simulink model "DriverInLoopSpeedgoat"  (R2020b)
settings: Solver=ode3  StartTime=0.0  StopTime=inf  FixedStep=1e-3  RelTol=5e-3  EnableMultiTasking=on
StartFcn:
  | %tic
StopFcn:
  | %toc
model workspace (MAT data in the model file):
  A_mu = 10
  B_reff = 8.386
  Cz = 7766.25
  DCT_Param.Transmission.Ratios = [3.78 2.18 1.43 1.03 0.935 0.84]
  DCT_Param.Transmission.Shaft_Inertia_Odd = 0.0023
  DCT_Param.Transmission.Shaft_Inertia_Even = 0.0009
  DCT_Param.Transmission.Shaft_Inertia_Output = 0.008
  DCT_Param.Transmission.Gear_Inertia = 0.001
  DCT_Param.Transmission.Gear_Efficiency = 0.94
  DCT_Param.Transmission.Gear_Ang_Vel_Thr = 0.01
  DCT_Param.Transmission.Shaft_Velocity_Odd = 0
  DCT_Param.Transmission.Shaft_Velocity_Even = 0
  DCT_Param.Transmission.Shaft_Velocity_Output = 0
  DCT_Param.Transmission.Gear_Initial_Velocity = 0
  DCT_Param.Transmission.Abstract.Compliance = 100000
  DCT_Param.Transmission.Abstract.Damping = 10000
  DCT_Param.Transmission.Abstract.Ratio_Time_Const = 0.05
  DCT_Param.Transmission.Abstract.Shift_Gear_Delay = 25
  DCT_Param.Clutch.Torque_Radius = 130
  DCT_Param.Clutch.Num_Friction_Surfaces = 4
  DCT_Param.Clutch.Engagement_Piston_Area = 0.001
  DCT_Param.Clutch.Kinetic_Friction_Coeff = 0.3
  DCT_Param.Clutch.Static_Friction_Coeff = 0.31
  DCT_Param.Clutch.Derating_Factor = 1
  DCT_Param.Clutch.Clutch_Velocity_Tolerance = 0.001
  DCT_Param.Clutch.Threshold_Pressure = 1
  DCT_Param.Clutch.Drag_Torque_Coeff = 0
  DCT_Param.Dog_Clutch.Max_Torque = 1000
  DCT_Param.Dog_Clutch.Teeth_Mean_Radius = 50
  DCT_Param.Dog_Clutch.Tooth_Height = 10
  DCT_Param.Dog_Clutch.Ring_Hub_Clearance = 3
  DCT_Param.Dog_Clutch.Ring_Stop_Stiffness = 1000000
  DCT_Param.Dog_Clutch.Ring_Stop_Damping = 1000
  DCT_Param.Dog_Clutch.Shift_Linkage_Damping = 100
  DCT_Param.Dog_Clutch.Max_Engage_Velocity = 1000000
  DCT_Param.Dog_Clutch.Tooth_Engage_Overlap = 3
  DCT_Param.Vehicle.Mass = 1600
  DCT_Param.Vehicle.Wheels_Per_Axle = 2
  DCT_Param.Vehicle.Distance_CG_FrontAxle = 1.7
  DCT_Param.Vehicle.Distance_CG_RearAxle = 2
  DCT_Param.Vehicle.Distance_CG_Ground = 0.5
  DCT_Param.Vehicle.Frontal_Area = 3
  DCT_Param.Vehicle.Aero_Drag_Coeff = 0.4
  DCT_Param.Vehicle.Initial_Velocity = 0
  DCT_Param.Vehicle.Final_Drive_Ratio = 3.7
  DCT_Param.Vehicle.Final_Drive_Efficiency = 0.86
  DCT_Param.Vehicle.Final_Drive_Vel_Thresh = 0.01
  DCT_Param.Vehicle.Side_Shaft_Inertia = 0.01
  DCT_Param.Vehicle.Side_Shaft_Initial_Velocity = 0
  DCT_Param.Vehicle.Tire.Radius = 0.312
  DCT_Param.Vehicle.Tire.Inertia = 0.5
  DCT_Param.Vehicle.Tire.Initial_Velocity = 0
  DCT_Param.Vehicle.Tire.Slip_Vel_Thresh = 0.1
  DCT_Param.Vehicle.Tire.Nominal_Vertical_Load = 4000
  DCT_Param.Vehicle.Tire.C_Coeff = 1.685
  DCT_Param.Vehicle.Tire.D_Coeff = [1.21 -0.037]
  DCT_Param.Vehicle.Tire.E_Coeff = [0.344 0.095 -0.02 0]
  DCT_Param.Vehicle.Tire.BCD_Coeff = [21.51 -0.163 0.245]
  DCT_Param.Vehicle.Tire.H_Coeff = [-0.002 0.002]
  DCT_Param.Vehicle.Tire.V_Coeff = [0 0]
  DCT_Param.ICE.Max_Power = 100000
  DCT_Param.ICE.Speed_At_Max_Power = 5500
  DCT_Param.ICE.Max_Speed = 7000
  DCT_Param.ICE.Stall_Speed = 200
  DCT_Param.ICE.Shaft_Inertia = 0.2
  DCT_Param.ICE.Initial_Velocity = 800
  DCT_Param.ICE.Idle_Ref_Spd = 800
  DCT_Param.ICE.Engine_Time_Constant = 0.2
  DCT_Param.ICE.Initial_Normalized_Throttle = 0
  DCT_Param.ICE.Speed_Threshold = 20
  DCT_Param.ICE.FC.Speed_Vector = [0 368.421052632 736.842105263 1105.26315789 1473.68421053 1842.10526316 2210.52631579 2578.94736842 2947.36842105 3315.78947368 3684.21052632 4052.63157895 4421.05263158 4789.47368421 5157.89473684 5526.31578947 5894.73684211 6263.15789474 6631.57894737 7000]
  DCT_Param.ICE.FC.Torque_Vector = [0 10.5263157895 21.0526315789 31.5789473684 42.1052631579 52.6315789474 63.1578947368 73.6842105263 84.2105263158 94.7368421053 105.263157895 115.789473684 126.315789474 136.842105263 147.368421053 157.894736842 168.421052632 178.947368421 189.473684211 200]
  DCT_Param.ICE.FC.Consumption_Table = [0.262945178015 0.225304787522 0.201465019624 0.191425874321 0.195187351614 0.212749451502 0.244112173984 0.289275519063 0.348239486736 0.421004077004 0.507569289868 0.607935125326 ... (400 elements, 20x20)]
  DCT_Param.Shift_Map_Example.Pedal_Positions = [0.1 0.4 0.5 0.9]
  DCT_Param.Shift_Map_Example.Upshift_Speeds = [11  20  26  34.5  43; 14  26  35  44.5  55; 17  31  42  52.5  65; 21  39  52  66.5  80]
  DCT_Param.Shift_Map_Example.Downshift_Speeds = [8.9  17  23.6  32.4  40.8; 11.5  22.7  32  41.6  52.2; 14  27  38.1  50  62; 18  33  48  62.6  76.2]
  DCT_Param.Shift_Map_ORIG.Pedal_Positions = [0.1 0.4 0.5 0.9]
  DCT_Param.Shift_Map_ORIG.Upshift_Speeds = [11.5  23.5  35.5  45.5  55.5; 14.5  26.5  38.5  48.5  58.5; 17.5  29.5  41.5  51.5  61.5; 20.5  32.5  44.5  54.5  64.5]
  DCT_Param.Shift_Map_ORIG.Downshift_Speeds = [8.5  20.5  32.5  42.5  52.5; 11.5  23.5  35.5  45.5  55.5; 14.5  26.5  38.5  48.5  58.5; 17.5  29.5  41.5  51.5  61.5]
  DCT_Param.Shift_Map_OPT.Pedal_Positions = [0.1 0.4 0.5 0.9]
  DCT_Param.Shift_Map_OPT.Upshift_Speeds = [17.8469  29.8469  35.8159  41.2981  46.3004; 19.2469  33.9778  43.9778  53.9778  63.9778; 24.5469  41.9778  62.1778  78.5778  106.9778; 27.5469  59.3778  99.0445  109.0445  119.0445]
  DCT_Param.Shift_Map_OPT.Downshift_Speeds = [14.8469  26.8469  32.8159  38.2981  43.3004; 16.2469  30.9778  40.9778  50.9778  60.9778; 21.5469  38.9778  59.1778  75.5778  103.9778; 24.5469  56.3778  96.0445  106.0445  116.0445]
  DCT_Param.Shift_Map.Pedal_Positions = [0.1 0.4 0.5 0.9]
  DCT_Param.Shift_Map.Upshift_Speeds = [11.5  23.5  35.5  45.5  55.5; 14.5  26.5  38.5  48.5  58.5; 17.5  29.5  41.5  51.5  61.5; 20.5  32.5  44.5  54.5  64.5]
  DCT_Param.Shift_Map.Downshift_Speeds = [8.5  20.5  32.5  42.5  52.5; 11.5  23.5  35.5  45.5  55.5; 14.5  26.5  38.5  48.5  58.5; 17.5  29.5  41.5  51.5  61.5]
  DCT_Param.Control.Clutch.Min_Lock_Pressure = 2000000
  DCT_Param.Control.Clutch.Max_Lock_Pressure = 5000000
  DCT_Param.Control.Clutch.Max_Unlock_Pressure = 500000
  DCT_Param.Control.Engine_Start_RPM = 800
  DCT_Param.Control.Engine_Stop_RPM = 790
  DCT_Param.Control.Mode_Logic_TS = 0.1
  DCT_Param.Control.ICE.Kp = 0.02
  DCT_Param.Control.ICE.Ki = 0.01
  DCT_Param.Control.Gen.Kp = 10
  DCT_Param.Control.Gen.Ki = 3
  DCT_Param.Control.Mot.Kp = 500
  DCT_Param.Control.Mot.Ki = 300
  DCT_Param.Control.Veh_Spd.Kp = 0.02
  DCT_Param.Control.Veh_Spd.Ki = 0.04
  DCT_Param.Driver.Kp = 400
  DCT_Param.Driver.Ki = 0.001
  DCT_Param.Driver.Pedal_Filter_Const = 0.01
  DCT_Param.Dog_Clutches.Pulse_Delay = 50
  DCT_Param.Dog_Clutches.Pulse_Length = 20
  DCT_Param.Animation.Teeth_Ratios = [0.338461538462 0.555555555556 0.916666666667 0.96 1.17948717949 1.92307692308]
  DCT_Param.Animation.Teeth_Ratios_Reverse = [0.458333333333 0.75]
  DCT_Param.Shift_Map_OPT506.Pedal_Positions = [0.1 0.4 0.5 0.9]
  DCT_Param.Shift_Map_OPT506.Upshift_Speeds = [18  30.2  48.3  67.3322  77.3429; 20.1  36.85  66.6178  76.7537  86.7537; 21.1  40.25  71.0189  81.0189  91.7873; 24.1  63.75  80.7523  105.9489  115.9489]
  DCT_Param.Shift_Map_OPT506.Downshift_Speeds = [15  27.2  45.3  64.3322  74.3429; 17.1  33.85  63.6178  73.7537  83.7537; 18.1  37.25  68.0189  78.0189  88.7873; 21.1  60.75  77.7523  102.9489  112.9489]
  DCT_Param.Shift_Map_OPTAbsRea176.Pedal_Positions = [0.1 0.4 0.5 0.9]
  DCT_Param.Shift_Map_OPTAbsRea176.Upshift_Speeds = [17.8469  29.8469  35.7875  44.0901  49.4243; 18.9219  34.1312  45.8256  59.7585  69.7585; 32.1719  43.4585  53.51  103.2151  114.6401; 35.1719  59.2585  99.5217  109.5217  119.5217]
  DCT_Param.Shift_Map_OPTAbsRea176.Downshift_Speeds = [14.8469  26.8469  32.7875  41.0901  46.4243; 15.9219  31.1312  42.8256  56.7585  66.7585; 29.1719  40.4585  50.51  100.2151  111.6401; 32.1719  56.2585  96.5217  106.5217  116.5217]
  DLC_XEnd = 236.9
  DLC_XStart = 175.9
  DLC_YStart = 3.2153
  D_reff = 0.25826
  Downshift_Speeds = [9.5625  23.0625  36.5625  47.8125; 12.9375  26.4375  39.9375  51.1875; 16.3125  29.8125  43.3125  54.5625; 19.6875  33.1875  46.6875  57.9375]
  EngRevLim = 7000
  Pedal_Positions = [0.1 0.4 0.5 0.9]
  SUS.Stiffness = 24000
  SUS.Damping.Constant = 1262
  SUS.Damping.Rebound = [4040 4950 2883 2043]
  SUS.Damping.Compression = [3600 3420 1863 1472]
  SUS.PistonSpeed = [0.05 0.1 0.3 0.6]
  SUS.UnsprungMass.Fr = 21.0693333333
  SUS.UnsprungMass.Rr = 21.0693333333
  Upshift_Speeds = [12.9375  26.4375  39.9375  51.1875; 16.3125  29.8125  43.3125  54.5625; 19.6875  33.1875  46.6875  57.9375; 33  52.5  77.25  100.5]
  VEH.Mass = 1181
  VEH.StaticNormalFrontLoad.FR = 264.666666667
  VEH.StaticNormalFrontLoad.FL = 264.666666667
  VEH.StaticNormalRearLoad.RR = 322
  VEH.StaticNormalRearLoad.RL = 322
  VEH.WheelBase = 3.075
  VEH.FrontAxlePositionfromCG = 1.515
  VEH.RearAxlePositionfromCG = 1.504
  VEH.HeightCG = 0.134
  VEH.FrontalArea = 2.11
  VEH.DragCoefficient = 0.33
  VEH.NumberOfWheelsPerAxle = 2
  VEH.Thread.FR = 1.705
  VEH.Thread.RR = 1.705
  VEH.PitchMomentInertia = 1922.66666667
  VEH.RollMomentInertia = 432.333333333
  VEH.YawMomentInertia = 2066
  VEH.SteeringRatio = 18
  VEH.TrackWidth = 1.922
  VEH.SprungMass = 1096.72266667
  VEH.InitialLongPosition = -26
  VEH.InitialLatPosition = 76
  VEH.InitialVertPosition = 0
  VEH.InitialRollAngle = 0
  VEH.InitialPitchAngle = 0
  VEH.InitialYawAngle = -0.698131700798
  VEH.InitialLongVel = 0
  VEH.InitialLatVel = 0
  VEH.InitialVertVel = 0
  VEH.InitialRollRate = 0
  VEH.InitialPitchRate = 0
  VEH.InitialYawRate = 0
  V_o = 16.7
  V_xlow = 1
  WH.Tire.Radius.Front = 0.384
  WH.Tire.Radius.Rear = 0.401
  WH.Tire.Sidewall = 0.245
  WH.Tire.RollingResistCoeff = 0.0103
  WH.Tire.Magic.B = 10
  WH.Tire.Magic.C = 1.9
  WH.Tire.Magic.D = 1
  WH.Tire.Magic.E = 0.97
  WH.Tire.Magic.Bx = 12
  WH.Tire.Magic.Cx = 1.9
  WH.Tire.Magic.Dx = 0.72
  WH.Tire.Magic.Ex = 0.95
  WH.Tire.Magic.By = 12
  WH.Tire.Magic.Cy = 1.3
  WH.Tire.Magic.Dy = 0.75
  WH.Tire.Magic.Ey = 0.2
  WH.Tire.Front.Ky = 40000
  WH.Tire.Rear.Ky = 40000
  WH.Tire.Kz = 320000
  WH.Tire.Damping = 100
  WH.Inertia = 1.00333333333
  WH.Mass = 11.4333333333
  WH.DampingCoefficient = 0.01
  WH.VelocityTol = 0.1
  a = 1.4
  alpha_max = 1.5
  alpha_min = -1.5
  b = 1.8
  c_zo = 209651
  epsilon = 0.1
  h = 0.134
  path.ISO3888p2.x = [0 2 12 25.5 36.5 49 61]
  path.ISO3888p2.y = [0 0 0 3.725 3.725 0 0]
  path.ISO3888p2.ylb = [1.225 1.225 1.225 4.725 4.725 1.5 1.5]
  path.ISO3888p2.yrb = [-1.225 -1.225 -1.225 2.225 2.225 -1.5 -1.5]
  path.CUSC.x = [10.668 21.336 36.576 54.864 73.152]
  path.CUSC.y = [0 0 5.1816 0 0]
  path.CUSC.ylb = [1.2192 1.2192 7.0104 1.8288 1.8288]
  path.CUSC.yrb = [-1.2192 -1.2192 3.3528 -1.8288 -1.8288]
  pio = 220000
  q_Fcx = 0
  q_Fz2 = 15.4
  q_Fzy = 0
  q_reo = 0.9974
  q_sx1 = -0.007764
  q_sx10 = 0.2824
  q_sx11 = 5.349
  q_sx12 = 0
  q_sx13 = 0
  q_sx14 = 0
  q_sx2 = 1.1915
  q_sx3 = 0.013948
  q_sx4 = 4.912
  q_sx5 = 1.02
  q_sx6 = 22.83
  q_sx7 = 0.7104
  q_sx8 = -0.023393
  q_sx9 = 0.6581
  q_sy1 = 0.00702
  q_sy2 = 0
  q_sy3 = 0.001515
  q_sy4 = 8.514e-05
  q_sy5 = 0
  q_sy6 = 0
  q_sy7 = 0.9008
  q_sy8 = -0.4089
  q_v1 = 0.0007742
  q_v2 = 0.04667
  r_Bx1 = 12.531
  r_Bx2 = 9.532
  r_Bx3 = 0
  r_By1 = 10.615
  r_By2 = 7.705
  r_By3 = 3.433e-06
  r_By4 = 0
  r_Cx1 = 1.019
  r_Cy1 = 1.0585
  r_Ex1 = -0.4487
  r_Ex2 = -0.4726
  r_Ey1 = 0.3132
  r_Ey2 = 7.63e-06
  r_Hx1 = 0.0002374
  r_Hy1 = 0.011646
  r_Hy2 = 7.63e-06
  r_Vy1 = 0.05654
  r_Vy2 = 7.63e-06
  r_Vy3 = 0
  r_Vy4 = 99.9
  r_Vy5 = 2
  r_Vy6 = 15.814
  r_o = 0.3135
  vehWidth = 2
  w = 1
  xdot_ref = 13.4112
libraries: autolibutils x7, simulink x6, slrealtimeutilitieslib x3, slrealtimeiplib x3, slrealtimeobsoletelib x1, dspstat3 x1
(part 1 of 2)
settings Model: SimulationMode=external  Creator=The MathWorks, Inc.  LastModifiedBy=timo.straessle
settings SolverCC: ConcurrentTasks=on  ZeroCrossAlgorithm=Adaptive  PositivePriorityOrder=on  AutoInsertRateTranBlk=on  InsertRTBMode=Never (minimum delay)  DecoupledContinuousIntegration=on  MinimalZcImpactIntegration=on
settings DataIOCC: SaveFormat=StructureWithTime
settings OptimizationCC: BlockReduction=off  OptimizeBlockIOStorage=off  BufferReuse=off  GlobalBufferReuse=off  ExpressionFolding=off  LocalBlockOutputs=off  OptimizeDataStoreBuffers=off  BusAssignmentInplaceUpdate=off
settings DebuggingCC: SignalInfNanChecking=error  ArtificialAlgebraicLoopMsg=none  IgnoredZcDiagnostic=none  InheritedTsInSrcMsg=none  TasksWithSamePriorityMsg=none  SigSpecEnsureSampleTimeMsg=none  ModelReferenceSymbolNameMessage=none  ModelReferenceExtraNoncontSigs=none  ArithmeticOperatorsInVariantConditions=warning
settings HardwareCC: ProdBitPerLong=64  ProdLongLongMode=on  ProdHWDeviceType=Intel->x86-64 (Linux 64)
settings ModelReferenceCC: UpdateModelReferenceTargets=IfOutOfDate  ModelReferenceMinAlgLoopOccurrences=on  PropagateSignalLabelsOutOfModel=off
settings SFSimCC: SimUseLocalCustomCode=off  CustomCodeUndefinedFunction=UseInterfaceOnly
settings RTWCC: Description=Simulink Real-Time  SystemTargetFile=slrealtime.tlc  TemplateMakefile=slrealtime_default_tmf  RTWUseLocalCustomCode=off  Toolchain=Simulink Real-Time Toolchain  BuildConfiguration=Faster Runs  CodeExecutionProfiling=on  TargetLang=C++

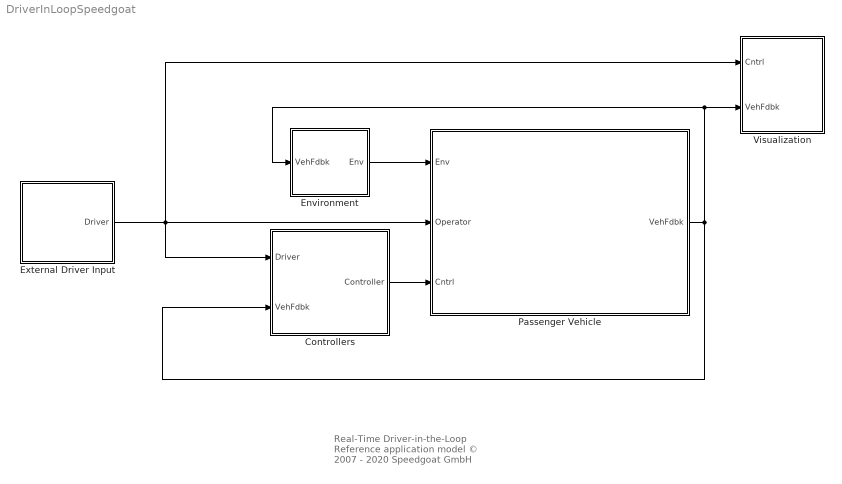
== system DriverInLoopSpeedgoat ==
  note: Real-Time Driver-in-the-Loop
      |
      | Reference application model
      | © 2007 - 2020 Speedgoat GmbH
  Controllers : Subsystem
      mask Display: image('SystemControllers.png')
  Environment : Subsystem
      mask Display: disp('Environment')
  External Driver Input : Subsystem  Variant=on  VariantControlMode=label  LabelModeActiveChoice=G29 connected to Host
      mask Display: image('driverlatlong.png');
  Passenger Vehicle : Subsystem
      mask Display: image('PassengerVehicle.png')
  Visualization : Subsystem
      mask Display: disp('Visualization')
  wires:
  Passenger Vehicle/1(VehFdbk) -> Controllers/2(VehFdbk), Environment/1(VehFdbk), Visualization/2(VehFdbk)
  Controllers/1(Controller) -> Passenger Vehicle/3(Cntrl)
  Environment/1(Env) -> Passenger Vehicle/1(Env)
  External Driver Input/1(Driver) -> Visualization/1(Cntrl), Controllers/1(Driver), Passenger Vehicle/2(Operator)

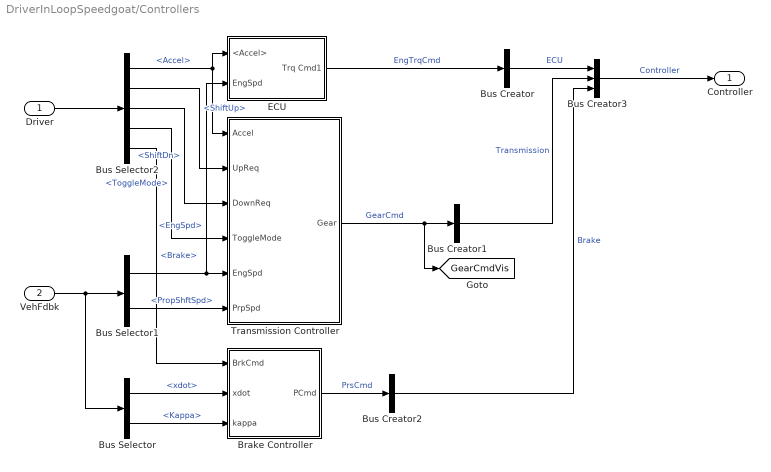
== system DriverInLoopSpeedgoat/Controllers ==
  Driver : Inport
  VehFdbk : Inport  Port=2
  Brake Controller : Subsystem
  Bus Creator : BusCreator  Inputs=1
  Bus Creator1 : BusCreator  Inputs=1
  Bus Creator2 : BusCreator  Inputs=1
  Bus Creator3 : BusCreator  Inputs=3
  Bus Selector : BusSelector  OutputSignals=Body.xdot,Wheels.Kappa
  Bus Selector1 : BusSelector  OutputSignals=Driveline.EngSpd,Driveline.PropShftSpd
  Bus Selector2 : BusSelector  OutputSignals=Accel,ShiftUp,ShiftDn,ToggleMode,Brake
  ECU : Subsystem
  Transmission Controller : Subsystem
  Controller : Outport  VectorParamsAs1DForOutWhenUnconnected=off
  tag scope: GearCmdVis=global
  wires:
  Brake Controller/1(PCmd) -> Bus Creator2/1  "PrsCmd"
  Bus Creator3/1 -> Controller/1  "Controller"
  Bus Creator2/1 -> Bus Creator3/3  "Brake"
  Bus Creator/1 -> Bus Creator3/1  "ECU"
  Driver/1 -> Bus Selector2/1
  Transmission Controller/1(Gear) -> Bus Creator1/1, [GearCmdVis]  "GearCmd"
  Bus Selector1/2 -> Transmission Controller/6(PrpSpd)  "<PropShftSpd>"
  Bus Selector2/5 -> Brake Controller/1(BrkCmd)  "<Brake>"
  VehFdbk/1 -> Bus Selector1/1, Bus Selector/1
  Bus Selector/1 -> Brake Controller/2(xdot)  "<xdot>"
  Bus Selector2/1 -> ECU/1(<Accel>), Transmission Controller/1(Accel)  "<Accel>"
  Bus Selector/2 -> Brake Controller/3(kappa)  "<Kappa>"
  ECU/1(Trq Cmd1) -> Bus Creator/1  "EngTrqCmd"
  Bus Creator1/1 -> Bus Creator3/2  "Transmission"
  Bus Selector1/1 -> Transmission Controller/5(EngSpd), ECU/2(EngSpd)  "<EngSpd>"
  Bus Selector2/2 -> Transmission Controller/2(UpReq)  "<ShiftUp>"
  Bus Selector2/3 -> Transmission Controller/3(DownReq)  "<ShiftDn>"
  Bus Selector2/4 -> Transmission Controller/4(ToggleMode)  "<ToggleMode>"

== system DriverInLoopSpeedgoat/Environment ==
  VehFdbk : Inport
  Bus Creator1 : BusCreator  Inputs=2
  Bus Creator3 : BusCreator  Inputs=2
  Constant3 : Constant  Value=0
  Constant4 : Constant  Value=0
  Constant5 : Constant  Value=0
  Friction Scaling : Subsystem  Variant=on  VariantControlMode=label  LabelModeActiveChoice=0
  Ground Height : Subsystem  Variant=on  VariantControlMode=label  LabelModeActiveChoice=1
  Vector Concatenate : Concatenate  NumInputs=3
  Env : Outport  VectorParamsAs1DForOutWhenUnconnected=off
  wires:
  Friction Scaling/1(mu) -> Bus Creator3/2  "mu"
  Constant5/1 -> Vector Concatenate/3  "Z"
  Vector Concatenate/1 -> Bus Creator1/1  "Wind"
  Constant3/1 -> Vector Concatenate/1  "X"
  Constant4/1 -> Vector Concatenate/2  "Y"
  Bus Creator3/1 -> Bus Creator1/2  "Gnd"
  Bus Creator1/1 -> Env/1
  VehFdbk/1 -> Friction Scaling/1(VehFdbk)
  Ground Height/1(z) -> Bus Creator3/1

== system DriverInLoopSpeedgoat/External Driver Input ==
  note: 1) Add Subsystem or Model blocks as valid variant choices.
      | 2) You cannot connect blocks at this level. At simulation, connectivity is automatically
      | determined, based on the active variant and port name matching.
  External Driver - Host : Subsystem  VariantControl=G29 connected to Host
      mask Display: image('driverlatlong.png');
  External Driver - Speedgoat : Subsystem  TreatAsAtomicUnit=on  VariantControl=G20 connected to Speedgoat  mask{selection=LogitechG920}
      mask prompts: selection "Select External Steering Device:"
      settings: MinAlgLoopOccurrences=on
      mask TypeOptions selection: LogitechG920 | LogitechF310 | ThrustmasterT150 | FanatecClubSport
      mask Callback selection:
      | % set variant for Axes mapping
      | set_param([gcb, '/MapAndScaleAxes'],...
      |           'OverrideUsingVariant', get_param(gcb, 'selection'));
      | 
      | % set variant for Button mapping
      | set_param([gcb, '/MapButtons'],...
      |           'OverrideUsingVariant', get_param(gcb, 'selection'));
      mask Display: image('driverlatlong.png');
  Driver : Outport

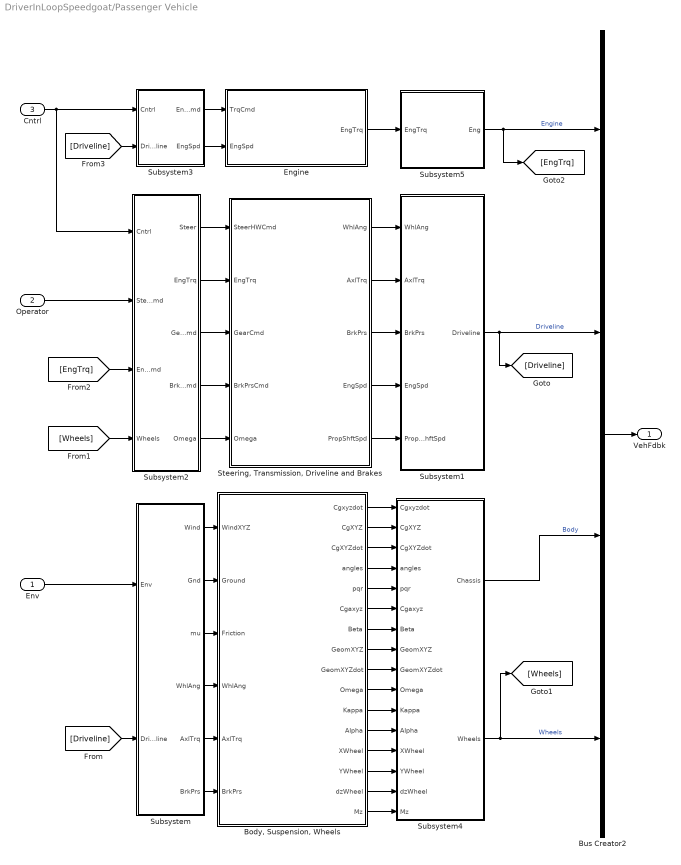
== system DriverInLoopSpeedgoat/Passenger Vehicle ==
  Env : Inport
  Operator : Inport  Port=2
  Cntrl : Inport  Port=3
  "Body, Suspension, Wheels" : Subsystem  Variant=on  VariantControlMode=label  LabelModeActiveChoice=3
  Bus Creator2 : BusCreator  Inputs=4
  Engine : Subsystem  Variant=on  VariantControlMode=label  LabelModeActiveChoice=0
  "Steering, Transmission, Driveline and Brakes" : Subsystem  Variant=on  VariantControlMode=label  LabelModeActiveChoice=0
  Subsystem : Subsystem
  Subsystem1 : Subsystem
  Subsystem2 : Subsystem
  Subsystem3 : Subsystem
  Subsystem4 : Subsystem
  Subsystem5 : Subsystem
  VehFdbk : Outport  VectorParamsAs1DForOutWhenUnconnected=off
  wires:
  "Body, Suspension, Wheels"/9(GeomXYZdot) -> Subsystem4/9(GeomXYZdot)
  "Body, Suspension, Wheels"/11(Kappa) -> Subsystem4/11(Kappa)
  Subsystem4/2(Wheels) -> [Wheels], Bus Creator2/4  "Wheels"
  Subsystem/1(Wind) -> "Body, Suspension, Wheels"/1(WindXYZ)
  Engine/1(EngTrq) -> Subsystem5/1("EngTrq ")
  Subsystem2/2(EngTrq) -> "Steering, Transmission, Driveline and Brakes"/2(EngTrq)
  "Body, Suspension, Wheels"/12(Alpha) -> Subsystem4/12(Alpha)
  Env/1 -> Subsystem/1(Env)
  "Steering, Transmission, Driveline and Brakes"/3(BrkPrs) -> Subsystem1/3(BrkPrs)
  "Body, Suspension, Wheels"/14(YWheel) -> Subsystem4/14(YWheel)
  "Body, Suspension, Wheels"/1(Cgxyzdot) -> Subsystem4/1(Cgxyzdot)
  "Body, Suspension, Wheels"/13(XWheel) -> Subsystem4/13(XWheel)
  Cntrl/1 -> Subsystem3/1(Cntrl), Subsystem2/1(Cntrl)
  "Body, Suspension, Wheels"/2(CgXYZ) -> Subsystem4/2(CgXYZ)
  "Body, Suspension, Wheels"/7(Beta) -> Subsystem4/7(Beta)
  "Body, Suspension, Wheels"/6(Cgaxyz) -> Subsystem4/6(Cgaxyz)
  "Steering, Transmission, Driveline and Brakes"/4(EngSpd) -> Subsystem1/4(EngSpd)
  "Body, Suspension, Wheels"/8(GeomXYZ) -> Subsystem4/8(GeomXYZ)
  Subsystem3/1(EngTrqCmd) -> Engine/1(TrqCmd)
  Subsystem/2(Gnd) -> "Body, Suspension, Wheels"/2(Ground)
  Subsystem5/1(Eng) -> [EngTrq], Bus Creator2/1  "Engine"
  [Driveline] -> Subsystem3/2(Driveline)
  [EngTrq] -> Subsystem2/3(EngTrqCmd)
  Bus Creator2/1 -> VehFdbk/1
  Subsystem2/4(BrkPrsCmd) -> "Steering, Transmission, Driveline and Brakes"/4(BrkPrsCmd)
  Subsystem2/5(Omega) -> "Steering, Transmission, Driveline and Brakes"/5(Omega)
  "Body, Suspension, Wheels"/3(CgXYZdot) -> Subsystem4/3(CgXYZdot)
  "Body, Suspension, Wheels"/15(dzWheel) -> Subsystem4/15(dzWheel)
  [Driveline] -> Subsystem/2(Driveline)
  Operator/1 -> Subsystem2/2(SteerCmd)
  [Wheels] -> Subsystem2/4(Wheels)
  Subsystem/5(AxlTrq) -> "Body, Suspension, Wheels"/5(AxlTrq)
  Subsystem1/1(Driveline) -> [Driveline], Bus Creator2/2  "Driveline"
  "Steering, Transmission, Driveline and Brakes"/2(AxlTrq) -> Subsystem1/2(AxlTrq)
  "Body, Suspension, Wheels"/4(angles) -> Subsystem4/4(angles)
  "Steering, Transmission, Driveline and Brakes"/5(PropShftSpd) -> Subsystem1/5(PropShftSpd)
  Subsystem/4(WhlAng) -> "Body, Suspension, Wheels"/4(WhlAng)
  Subsystem2/1(Steer) -> "Steering, Transmission, Driveline and Brakes"/1(SteerHWCmd)
  "Body, Suspension, Wheels"/5(pqr) -> Subsystem4/5(pqr)
  Subsystem3/2(EngSpd) -> Engine/2(EngSpd)
  "Steering, Transmission, Driveline and Brakes"/1(WhlAng) -> Subsystem1/1(WhlAng)
  Subsystem/6(BrkPrs) -> "Body, Suspension, Wheels"/6(BrkPrs)
  Subsystem2/3(GearCmd) -> "Steering, Transmission, Driveline and Brakes"/3(GearCmd)
  Subsystem/3(mu) -> "Body, Suspension, Wheels"/3(Friction)
  "Body, Suspension, Wheels"/10(Omega) -> Subsystem4/10(Omega)
  Subsystem4/1(Chassis) -> Bus Creator2/3  "Body"
  "Body, Suspension, Wheels"/16(Mz) -> Subsystem4/16(Mz)

== system DriverInLoopSpeedgoat/Visualization ==
  note: Vehicle Response
  note: Driver Commands
  Cntrl : Inport
  VehFdbk : Inport  Port=2
  Acceleration Cmd : LinearGaugeBlock  ScaleMax=1
  Brake Cmd : LinearGaugeBlock  ScaleMax=1
  Engine Tach [rpm] : CircularGaugeBlock  ScaleMax=8000  TickInterval=1000
  Handwheel Angle [deg] : SemiCircularGaugeBlock  ScaleMin=-300  ScaleMax=300  TickInterval=60
  Lateral Acceleration [g] : SemiCircularGaugeBlock  ScaleMin=-1  ScaleMax=1  TickInterval=0.5
  Speed [mph] : CircularGaugeBlock
  UDP Send : Subsystem
  wires:
  Cntrl/1 -> UDP Send/1(Cntrl)
  VehFdbk/1 -> UDP Send/2(VehFdbk)  "VehFdbk"

== system DriverInLoopSpeedgoat/Controllers/Brake Controller ==
  BrkCmd : Inport
  xdot : Inport  Port=2
  kappa : Inport  Port=3
  Abs : Abs  ZeroCross=off
  Bang Bang ABS : Subsystem  VariantControl=1
  Constant1 : Constant  Value=-20
  Gain3 : Gain
  Integrator2 : Integrator  LimitOutput=on  UpperSaturationLimit=1  LowerSaturationLimit=0
  Saturation : Saturate  UpperLimit=1  LowerLimit=0  ZeroCross=off
  Switch1 : Switch  Criteria=u2 > Threshold  Threshold=.1
  Vector Concatenate2 : Concatenate  NumInputs=4
  PCmd : Outport  VectorParamsAs1DForOutWhenUnconnected=off
  wires:
  Constant1/1 -> Switch1/3
  Gain3/1 -> Switch1/1
  Saturation/1 -> Bang Bang ABS/3(<Kappa>)  "Kappa"
  Bang Bang ABS/1(PCmd) -> PCmd/1
  kappa/1 -> Abs/1
  Integrator2/1 -> Vector Concatenate2/4, Vector Concatenate2/3, Vector Concatenate2/2, Vector Concatenate2/1
  xdot/1 -> Bang Bang ABS/2(xdot)
  Abs/1 -> Saturation/1
  Vector Concatenate2/1 -> Bang Bang ABS/1(Pref)  "Reference P"
  BrkCmd/1 -> Switch1/2, Gain3/1
  Switch1/1 -> Integrator2/1

== system DriverInLoopSpeedgoat/Controllers/ECU ==
  <Accel> : Inport
  EngSpd : Inport  Port=2
  Acc to Torque Request : Gain  Gain=150
  Rev Limiter Control : Subsystem
  Signal Specification : SignalSpecification  Unit=rpm
  Unit Conversion : UnitConversion
  Trq Cmd1 : Outport  VectorParamsAs1DForOutWhenUnconnected=off
  wires:
  <Accel>/1 -> Acc to Torque Request/1
  Signal Specification/1 -> Rev Limiter Control/2(EngSpd)  "EngSpd"
  Unit Conversion/1 -> Signal Specification/1
  EngSpd/1 -> Unit Conversion/1
  Acc to Torque Request/1 -> Rev Limiter Control/1(TrqCmd)
  Rev Limiter Control/1(TrqCmdRevLimited) -> Trq Cmd1/1

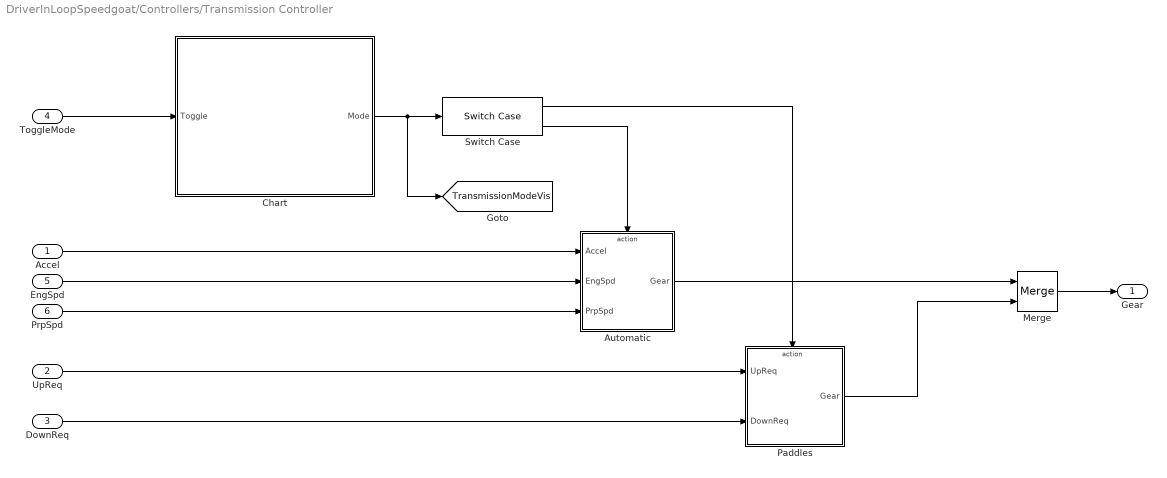
== system DriverInLoopSpeedgoat/Controllers/Transmission Controller ==
  Accel : Inport
  UpReq : Inport  Port=2
  DownReq : Inport  Port=3
  ToggleMode : Inport  Port=4
  EngSpd : Inport  Port=5
  PrpSpd : Inport  Port=6
  Automatic : Subsystem  TreatAsAtomicUnit=on
  Chart : Stateflow chart  TreatAsAtomicUnit=on
  Merge : Merge  InitialOutput=0
  Paddles : Subsystem  TreatAsAtomicUnit=on
  Switch Case : SwitchCase  CaseConditions={0,1}  ShowDefaultCase=off
  Gear : Outport
  tag scope: TransmissionModeVis=global
  wires:
  Chart/1(Mode) -> [TransmissionModeVis], Switch Case/1
  Switch Case/2 -> Automatic/Action
  Switch Case/1 -> Paddles/Action
  Automatic/1(Gear) -> Merge/1
  Paddles/1(Gear) -> Merge/2
  ToggleMode/1 -> Chart/1(Toggle)
  Merge/1 -> Gear/1
  Accel/1 -> Automatic/1(Accel)
  EngSpd/1 -> Automatic/2(EngSpd)
  PrpSpd/1 -> Automatic/3(PrpSpd)
  UpReq/1 -> Paddles/1(UpReq)
  DownReq/1 -> Paddles/2(DownReq)

== system DriverInLoopSpeedgoat/Environment/Friction Scaling ==
  note: 1) Add Subsystem or Model blocks as valid variant choices.
      | 2) You cannot connect blocks at this level. At simulation, connectivity is automatically
      | determined, based on the active variant and port name matching.
  VehFdbk : Inport
  Constant : Subsystem  VariantControl=0
  Lookup Table : Subsystem  VariantControl=1
  mu : Outport  VectorParamsAs1DForOutWhenUnconnected=off

== system DriverInLoopSpeedgoat/Environment/Ground Height ==
  note: 1) Add Subsystem or Model blocks as valid variant choices.
      | 2) You cannot connect blocks at this level. At simulation, connectivity is automatically
      | determined, based on the active variant and port name matching.
  3D Engine : Subsystem  VariantControl=1
  Constant : Subsystem  VariantControl=0
  z : Outport  VectorParamsAs1DForOutWhenUnconnected=off

== system DriverInLoopSpeedgoat/External Driver Input/External Driver - Host ==
  Abs : Abs
  Bus Creator1 : BusCreator  Inputs=7
  Data Type Conversion : DataTypeConversion  OutDataTypeStr=boolean
  Dead Zone : DeadZone  LowerValue=-0.04  UpperValue=0.04
  Dead Zone2 : DeadZone  LowerValue=-0.0078  UpperValue=0
  Ground : Ground
  Receive UDP : Subsystem  TreatAsAtomicUnit=on
  Saturation : Saturate  UpperLimit=1  LowerLimit=0
  Saturation1 : Saturate  UpperLimit=0  LowerLimit=-1
  Subsystem : Subsystem
  Wheel Angle Limit * Steer Ratio : Gain  Gain=450*pi/180
  Driver : Outport  VectorParamsAs1DForOutWhenUnconnected=off
  wires:
  Saturation/1 -> Bus Creator1/2  "Brake"
  Dead Zone/1 -> Wheel Angle Limit * Steer Ratio/1
  Saturation1/1 -> Abs/1
  Wheel Angle Limit * Steer Ratio/1 -> Bus Creator1/1  "SteerCmd"
  Ground/1 -> Bus Creator1/4  "Clutch"
  Bus Creator1/1 -> Driver/1  "Driver"
  Dead Zone2/1 -> Saturation1/1
  Abs/1 -> Bus Creator1/3  "Accel"
  Subsystem/2(AccelBrake) -> Dead Zone2/1, Saturation/1
  Subsystem/1(Steer) -> Dead Zone/1
  Subsystem/3(ShiftDn) -> Bus Creator1/5  "ShiftDn"
  Subsystem/4(ShiftUp) -> Bus Creator1/6  "ShiftUp"
  Receive UDP/2(Data) -> Subsystem/1(In1)
  Data Type Conversion/1 -> Subsystem/Enable
  Receive UDP/1(NumMsg) -> Data Type Conversion/1
  Subsystem/5(ToggleMode) -> Bus Creator1/7  "ToggleMode"

== system DriverInLoopSpeedgoat/External Driver Input/External Driver - Speedgoat ==
  Bus Creator : BusCreator  Inputs=2
  Bus Creator1 : BusCreator  Inputs=5
  Data Type Conversion : DataTypeConversion  OutDataTypeStr=double
  Data Type Conversion1 : DataTypeConversion  OutDataTypeStr=double
  MapAndScaleAxes : Subsystem  VariantControl=LogitechG920
  MapButtons : Subsystem  VariantControl=LogitechG920
  Mux : Mux  Inputs=2
  "Steering Wheel Read " : slrealtimeobsoletelib/Obsolete  ObsoleteBlock=logitechG29/Steering Wheel Read  ObsoleteParameters="MultiThreadCoSim:  auto sampleTime:  1e-3"  NumInports=0  NumOutports=5
      settings: SourceProductName=Simulink Real-Time
  Terminator : Terminator
  Terminator1 : Terminator
  Terminator2 : Terminator
  Driver : Outport  VectorParamsAs1DForOutWhenUnconnected=off
  wires:
  MapAndScaleAxes/4(Clutch) -> Bus Creator1/4  "Clutch"
  Bus Creator/1 -> Bus Creator1/5  "ShiftCmd"
  Bus Creator1/1 -> Driver/1
  MapAndScaleAxes/3(Brake) -> Bus Creator1/3  "Brake"
  MapAndScaleAxes/2(Accel) -> Bus Creator1/2  "Accel"
  MapAndScaleAxes/1(Steering) -> Bus Creator1/1  "Steer"
  "Steering Wheel Read "/4 -> Terminator/1
  "Steering Wheel Read "/5 -> Terminator1/1
  Mux/1 -> MapAndScaleAxes/1(WheelPedals)  "SteeringWheelAxes"
  "Steering Wheel Read "/3 -> Data Type Conversion1/1
  Data Type Conversion1/1 -> Mux/2
  "Steering Wheel Read "/2 -> Data Type Conversion/1
  Data Type Conversion/1 -> Mux/1
  "Steering Wheel Read "/1 -> MapButtons/1(Buttons)  "SteeringWheelButtons"
  MapButtons/1(LeftPaddle) -> Bus Creator/1  "ShiftDn"
  MapButtons/2(RightPaddle) -> Bus Creator/2  "ShiftUp"
  MapButtons/3(AllButtons) -> Terminator2/1

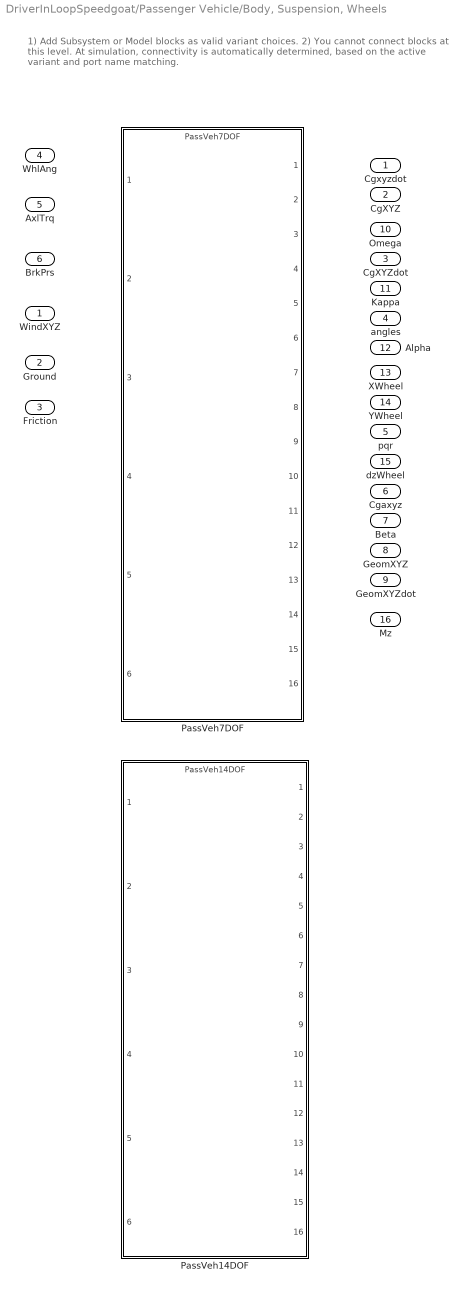
== system DriverInLoopSpeedgoat/Passenger Vehicle/Body, Suspension, Wheels ==
  note: 1) Add Subsystem or Model blocks as valid variant choices.
      | 2) You cannot connect blocks at this level. At simulation, connectivity is automatically
      | determined, based on the active variant and port name matching.
  WindXYZ : Inport
  Ground : Inport  Port=2  PortDimensions=4
  Friction : Inport  Port=3  PortDimensions=4
  WhlAng : Inport  Port=4
  AxlTrq : Inport  Port=5
  BrkPrs : Inport  Port=6
  PassVeh14DOF : ModelReference  DisableCoverage=on  ModelNameDialog=PassVeh14DOF  SimulationMode=Normal  VariantControl=3  ModelReferenceVersion=2.2
  PassVeh7DOF : ModelReference  DisableCoverage=on  ModelNameDialog=PassVeh7DOF  SimulationMode=Normal  VariantControl=1  ModelReferenceVersion=1.148
  Cgxyzdot : Outport  VectorParamsAs1DForOutWhenUnconnected=off
  CgXYZ : Outport  Port=2  VectorParamsAs1DForOutWhenUnconnected=off
  CgXYZdot : Outport  Port=3  VectorParamsAs1DForOutWhenUnconnected=off
  angles : Outport  Port=4  VectorParamsAs1DForOutWhenUnconnected=off
  pqr : Outport  Port=5  VectorParamsAs1DForOutWhenUnconnected=off
  Cgaxyz : Outport  Port=6  VectorParamsAs1DForOutWhenUnconnected=off
  Beta : Outport  Port=7  VectorParamsAs1DForOutWhenUnconnected=off
  GeomXYZ : Outport  Port=8  VectorParamsAs1DForOutWhenUnconnected=off
  GeomXYZdot : Outport  Port=9  VectorParamsAs1DForOutWhenUnconnected=off
  Omega : Outport  Port=10  PortDimensions=4  VectorParamsAs1DForOutWhenUnconnected=off
  Kappa : Outport  Port=11  PortDimensions=4  VectorParamsAs1DForOutWhenUnconnected=off
  Alpha : Outport  Port=12  PortDimensions=4  VectorParamsAs1DForOutWhenUnconnected=off
  XWheel : Outport  Port=13  VectorParamsAs1DForOutWhenUnconnected=off
  YWheel : Outport  Port=14  VectorParamsAs1DForOutWhenUnconnected=off
  dzWheel : Outport  Port=15  VectorParamsAs1DForOutWhenUnconnected=off
  Mz : Outport  Port=16  VectorParamsAs1DForOutWhenUnconnected=off

== system DriverInLoopSpeedgoat/Passenger Vehicle/Engine ==
  note: 1) Add Subsystem or Model blocks as valid variant choices.
      | 2) You cannot connect blocks at this level. At simulation, connectivity is automatically
      | determined, based on the active variant and port name matching.
  TrqCmd : Inport
  EngSpd : Inport  Port=2  Unit=rad/s
  Ideal Mapped Engine : ModelReference  DisableCoverage=on  ModelNameDialog=SiMappedEngineV  SimulationMode=Normal  VariantControl=0  ModelReferenceVersion=2.2
  EngTrq : Outport  VectorParamsAs1DForOutWhenUnconnected=off

== system DriverInLoopSpeedgoat/Passenger Vehicle/Steering, Transmission, Driveline and Brakes ==
  note: 1) Add Subsystem or Model blocks as valid variant choices.
      | 2) You cannot connect blocks at this level. At simulation, connectivity is automatically
      | determined, based on the active variant and port name matching.
  SteerHWCmd : Inport
  EngTrq : Inport  Port=2
  GearCmd : Inport  Port=3  OutDataTypeStr=int8
  BrkPrsCmd : Inport  Port=4  PortDimensions=4
  Omega : Inport  Port=5
  Driveline Ideal Fixed Gear : ModelReference  DisableCoverage=on  ModelNameDialog=Driveline  SimulationMode=Normal  VariantControl=0  ModelReferenceVersion=2.1
  WhlAng : Outport  VectorParamsAs1DForOutWhenUnconnected=off
  AxlTrq : Outport  Port=2  VectorParamsAs1DForOutWhenUnconnected=off
  BrkPrs : Outport  Port=3  PortDimensions=4  VectorParamsAs1DForOutWhenUnconnected=off
  EngSpd : Outport  Port=4  Unit=rad/s  VectorParamsAs1DForOutWhenUnconnected=off
  PropShftSpd : Outport  Port=5  VectorParamsAs1DForOutWhenUnconnected=off

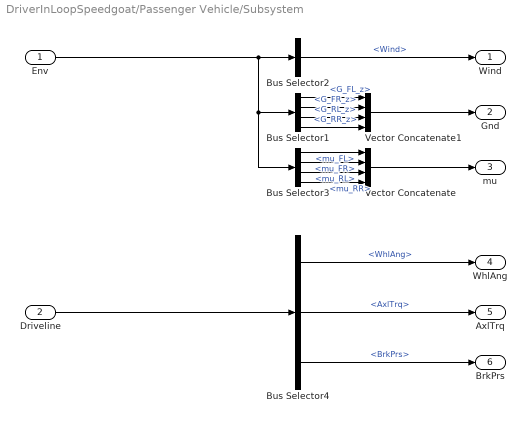
== system DriverInLoopSpeedgoat/Passenger Vehicle/Subsystem ==
  Env : Inport
  Driveline : Inport  Port=2
  Bus Selector1 : BusSelector  OutputSignals=Gnd.z.G_FL_z,Gnd.z.G_FR_z,Gnd.z.G_RL_z,Gnd.z.G_RR_z
  Bus Selector2 : BusSelector  OutputSignals=Wind
  Bus Selector3 : BusSelector  OutputSignals=Gnd.mu.mu_FL,Gnd.mu.mu_FR,Gnd.mu.mu_RL,Gnd.mu.mu_RR
  Bus Selector4 : BusSelector  OutputSignals=WhlAng,AxlTrq,BrkPrs
  Vector Concatenate : Concatenate  NumInputs=4
  Vector Concatenate1 : Concatenate  NumInputs=4
  Wind : Outport  VectorParamsAs1DForOutWhenUnconnected=off
  Gnd : Outport  Port=2  VectorParamsAs1DForOutWhenUnconnected=off
  mu : Outport  Port=3  VectorParamsAs1DForOutWhenUnconnected=off
  WhlAng : Outport  Port=4  VectorParamsAs1DForOutWhenUnconnected=off
  AxlTrq : Outport  Port=5  VectorParamsAs1DForOutWhenUnconnected=off
  BrkPrs : Outport  Port=6  VectorParamsAs1DForOutWhenUnconnected=off
  wires:
  Env/1 -> Bus Selector3/1, Bus Selector1/1, Bus Selector2/1
  Bus Selector2/1 -> Wind/1  "<Wind>"
  Bus Selector3/1 -> Vector Concatenate/1  "<mu_FL>"
  Bus Selector3/2 -> Vector Concatenate/2  "<mu_FR>"
  Bus Selector3/3 -> Vector Concatenate/3  "<mu_RL>"
  Bus Selector3/4 -> Vector Concatenate/4  "<mu_RR>"
  Vector Concatenate/1 -> mu/1
  Bus Selector1/1 -> Vector Concatenate1/1  "<G_FL_z>"
  Bus Selector1/2 -> Vector Concatenate1/2  "<G_FR_z>"
  Bus Selector1/3 -> Vector Concatenate1/3  "<G_RL_z>"
  Bus Selector1/4 -> Vector Concatenate1/4  "<G_RR_z>"
  Vector Concatenate1/1 -> Gnd/1
  Driveline/1 -> Bus Selector4/1
  Bus Selector4/2 -> AxlTrq/1  "<AxlTrq>"
  Bus Selector4/1 -> WhlAng/1  "<WhlAng>"
  Bus Selector4/3 -> BrkPrs/1  "<BrkPrs>"

== system DriverInLoopSpeedgoat/Passenger Vehicle/Subsystem1 ==
  WhlAng : Inport
  AxlTrq : Inport  Port=2
  BrkPrs : Inport  Port=3
  EngSpd : Inport  Port=4
  PropShftSpd : Inport  Port=5
  Bus Creator1 : BusCreator  Inputs=5
  Driveline : Outport  VectorParamsAs1DForOutWhenUnconnected=off
  wires:
  Bus Creator1/1 -> Driveline/1  "Driveline"
  PropShftSpd/1 -> Bus Creator1/5  "PropShftSpd"
  AxlTrq/1 -> Bus Creator1/2  "AxlTrq"
  WhlAng/1 -> Bus Creator1/1  "WhlAng"
  EngSpd/1 -> Bus Creator1/4  "EngSpd"
  BrkPrs/1 -> Bus Creator1/3  "BrkPrs"

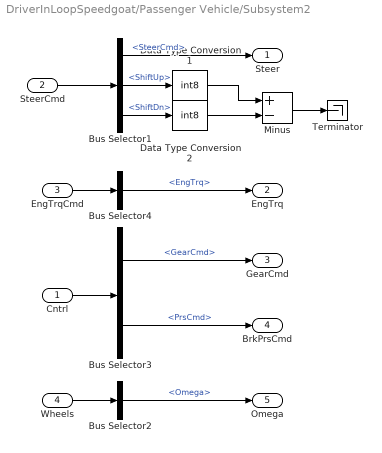
== system DriverInLoopSpeedgoat/Passenger Vehicle/Subsystem2 ==
  Cntrl : Inport
  SteerCmd : Inport  Port=2
  EngTrqCmd : Inport  Port=3
  Wheels : Inport  Port=4
  Bus Selector1 : BusSelector  OutputSignals=SteerCmd,ShiftUp,ShiftDn
  Bus Selector2 : BusSelector  OutputSignals=Omega
  Bus Selector3 : BusSelector  OutputSignals=Transmission.GearCmd,Brake.PrsCmd
  Bus Selector4 : BusSelector  OutputSignals=EngTrq
  Data Type Conversion1 : DataTypeConversion  OutDataTypeStr=int8
  Data Type Conversion2 : DataTypeConversion  OutDataTypeStr=int8
  Minus : Sum  Inputs=+-
  Terminator : Terminator
  Steer : Outport  VectorParamsAs1DForOutWhenUnconnected=off
  EngTrq : Outport  Port=2  VectorParamsAs1DForOutWhenUnconnected=off
  GearCmd : Outport  Port=3  VectorParamsAs1DForOutWhenUnconnected=off
  BrkPrsCmd : Outport  Port=4  VectorParamsAs1DForOutWhenUnconnected=off
  Omega : Outport  Port=5  VectorParamsAs1DForOutWhenUnconnected=off
  wires:
  Cntrl/1 -> Bus Selector3/1
  Bus Selector3/1 -> GearCmd/1  "<GearCmd>"
  SteerCmd/1 -> Bus Selector1/1
  Wheels/1 -> Bus Selector2/1
  Bus Selector2/1 -> Omega/1  "<Omega>"
  Bus Selector3/2 -> BrkPrsCmd/1  "<PrsCmd>"
  EngTrqCmd/1 -> Bus Selector4/1
  Bus Selector1/1 -> Steer/1  "<SteerCmd>"
  Bus Selector4/1 -> EngTrq/1  "<EngTrq>"
  Minus/1 -> Terminator/1
  Bus Selector1/2 -> Data Type Conversion1/1  "<ShiftUp>"
  Bus Selector1/3 -> Data Type Conversion2/1  "<ShiftDn>"
  Data Type Conversion1/1 -> Minus/1
  Data Type Conversion2/1 -> Minus/2

== system DriverInLoopSpeedgoat/Passenger Vehicle/Subsystem3 ==
  Cntrl : Inport
  Driveline : Inport  Port=2
  Bus Selector : BusSelector  OutputSignals=ECU.EngTrqCmd
  Bus Selector1 : BusSelector  OutputSignals=EngSpd
  EngTrqCmd : Outport  VectorParamsAs1DForOutWhenUnconnected=off
  EngSpd : Outport  Port=2  VectorParamsAs1DForOutWhenUnconnected=off
  wires:
  Driveline/1 -> Bus Selector1/1
  Cntrl/1 -> Bus Selector/1
  Bus Selector/1 -> EngTrqCmd/1  "<EngTrqCmd>"
  Bus Selector1/1 -> EngSpd/1  "<EngSpd>"

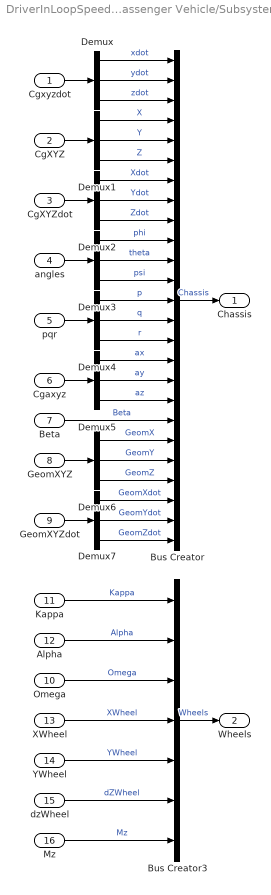
== system DriverInLoopSpeedgoat/Passenger Vehicle/Subsystem4 ==
  Cgxyzdot : Inport
  CgXYZ : Inport  Port=2
  CgXYZdot : Inport  Port=3
  angles : Inport  Port=4
  pqr : Inport  Port=5
  Cgaxyz : Inport  Port=6
  Beta : Inport  Port=7
  GeomXYZ : Inport  Port=8
  GeomXYZdot : Inport  Port=9
  Omega : Inport  Port=10
  Kappa : Inport  Port=11
  Alpha : Inport  Port=12
  XWheel : Inport  Port=13
  YWheel : Inport  Port=14
  dzWheel : Inport  Port=15
  Mz : Inport  Port=16
  Bus Creator : BusCreator  Inputs=25
  Bus Creator3 : BusCreator  Inputs=7
  Demux{,1..7} (8 alike) : Demux  Outputs=3
  Chassis : Outport  VectorParamsAs1DForOutWhenUnconnected=off
  Wheels : Outport  Port=2  VectorParamsAs1DForOutWhenUnconnected=off
  wires:
  Bus Creator/1 -> Chassis/1  "Chassis"
  Omega/1 -> Bus Creator3/3  "Omega"
  dzWheel/1 -> Bus Creator3/6  "dZWheel"
  Kappa/1 -> Bus Creator3/1  "Kappa"
  Bus Creator3/1 -> Wheels/1  "Wheels"
  YWheel/1 -> Bus Creator3/5  "YWheel"
  XWheel/1 -> Bus Creator3/4  "XWheel"
  Alpha/1 -> Bus Creator3/2  "Alpha"
  Cgxyzdot/1 -> Demux/1
  CgXYZ/1 -> Demux1/1
  CgXYZdot/1 -> Demux2/1
  angles/1 -> Demux3/1
  pqr/1 -> Demux4/1
  Cgaxyz/1 -> Demux5/1
  GeomXYZdot/1 -> Demux7/1
  GeomXYZ/1 -> Demux6/1
  Demux/1 -> Bus Creator/1  "xdot"
  Demux/2 -> Bus Creator/2  "ydot"
  Demux/3 -> Bus Creator/3  "zdot"
  Demux1/1 -> Bus Creator/4  "X"
  Demux1/2 -> Bus Creator/5  "Y"
  Demux1/3 -> Bus Creator/6  "Z"
  Demux2/1 -> Bus Creator/7  "Xdot"
  Demux2/2 -> Bus Creator/8  "Ydot"
  Demux2/3 -> Bus Creator/9  "Zdot"
  Demux3/1 -> Bus Creator/10  "phi"
  Demux3/2 -> Bus Creator/11  "theta"
  Demux3/3 -> Bus Creator/12  "psi"
  Demux4/1 -> Bus Creator/13  "p"
  Demux4/2 -> Bus Creator/14  "q"
  Demux4/3 -> Bus Creator/15  "r"
  Demux5/1 -> Bus Creator/16  "ax"
  Demux5/2 -> Bus Creator/17  "ay"
  Demux5/3 -> Bus Creator/18  "az"
  Beta/1 -> Bus Creator/19  "Beta"
  Demux6/1 -> Bus Creator/20  "GeomX"
  Demux6/2 -> Bus Creator/21  "GeomY"
  Demux6/3 -> Bus Creator/22  "GeomZ"
  Demux7/1 -> Bus Creator/23  "GeomXdot"
  Demux7/2 -> Bus Creator/24  "GeomYdot"
  Demux7/3 -> Bus Creator/25  "GeomZdot"
  Mz/1 -> Bus Creator3/7  "Mz"

== system DriverInLoopSpeedgoat/Passenger Vehicle/Subsystem5 ==
  "EngTrq " : Inport
  Bus Creator : BusCreator  Inputs=1
  Eng : Outport  VectorParamsAs1DForOutWhenUnconnected=off
  wires:
  "EngTrq "/1 -> Bus Creator/1  "EngTrq"
  Bus Creator/1 -> Eng/1

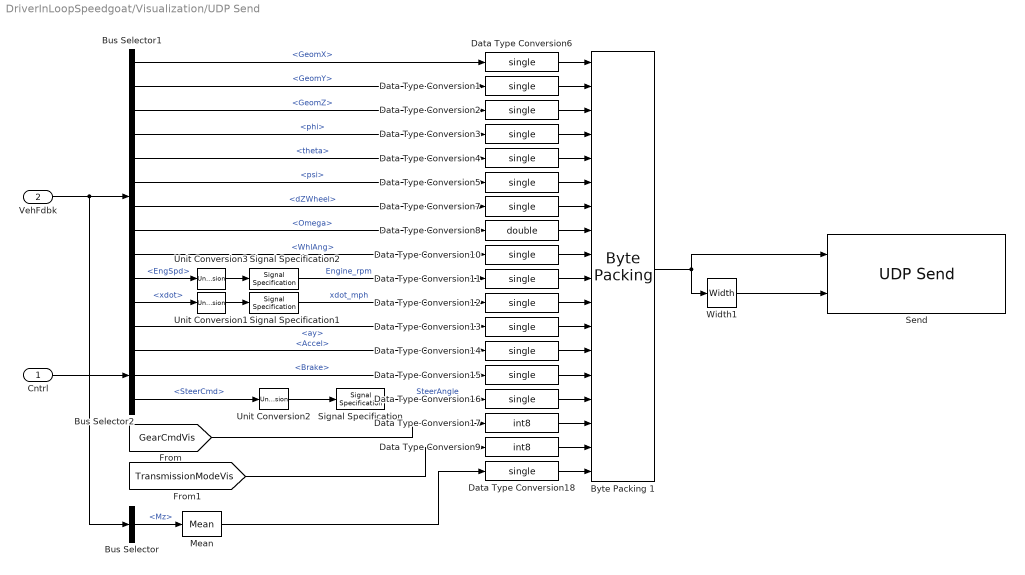
== system DriverInLoopSpeedgoat/Visualization/UDP Send ==
  Cntrl : Inport
  VehFdbk : Inport  Port=2
  Bus Selector : BusSelector  OutputSignals=Wheels.Mz
  Bus Selector1 : BusSelector  OutputSignals=Body.GeomX,Body.GeomY,Body.GeomZ,Body.phi,Body.theta,Body.psi,Wheels.dZWheel,Wheels.Omega,Driveline.WhlAng,Driveline.EngSpd,Body.xdot,Body.ay
  Bus Selector2 : BusSelector  OutputSignals=Accel,Brake,SteerCmd
  Byte Packing 1 : slrealtimeutilitieslib/Byte Packing  MaskPackedDataType=uint8  MaskUnpackedDataTypes={'single','single','single','single','single','single','single','double','single','single','single','single','single','single','single','int8','int8','single'}  MaskAlignment=1
  Data Type Conversion{1..7,10..16,18} (15 alike) : DataTypeConversion  OutDataTypeStr=single
  Data Type Conversion17 : DataTypeConversion  OutDataTypeStr=int8
  Data Type Conversion8 : DataTypeConversion  OutDataTypeStr=double
  Data Type Conversion9 : DataTypeConversion  OutDataTypeStr=int8
  Mean : dspstat3/Mean  run=off  InputProcessing=Columns as channels (frame based)  reset_popup=None  directionMode=Each column  dimension=1  roiEnable=off  roiType=Rectangles  roiPortion=Entire ROI  roiOutput=Individual statistics for each ROI  roiFlag=off  roundingMode=Floor  overflowMode=off  outputDataTypeStr=Inherit: Same as accumulator  outputMin=[]  outputMax=[]  outputLastDataTypeStr=Inherit: Same as accumulator
  Send : slrealtimeiplib/UDP Send  useHostTargetConn=on  ipAddress=target_ip  localPort=-1  toAddress=host_ip  toPort=25001  sampleTime=1e-3
      settings: SourceProductBaseCode=XP
  Signal Specification : SignalSpecification  Unit=deg
  Signal Specification1 : SignalSpecification  Unit=mph
  Signal Specification2 : SignalSpecification  Unit=rpm
  Unit Conversion1 : UnitConversion
  Unit Conversion2 : UnitConversion
  Unit Conversion3 : UnitConversion
  Width1 : Width
  wires:
  Bus Selector1/11 -> Unit Conversion1/1  "<xdot>"
  Signal Specification2/1 -> Data Type Conversion11/1  "Engine_rpm"
  Unit Conversion3/1 -> Signal Specification2/1
  Bus Selector2/1 -> Data Type Conversion14/1  "<Accel>"
  Bus Selector1/12 -> Data Type Conversion13/1  "<ay>"
  Data Type Conversion3/1 -> Byte Packing 1/4
  Byte Packing 1/1 -> Send/1, Width1/1
  Data Type Conversion1/1 -> Byte Packing 1/2
  Data Type Conversion8/1 -> Byte Packing 1/8
  VehFdbk/1 -> Bus Selector1/1, Bus Selector/1
  Unit Conversion2/1 -> Signal Specification/1
  Signal Specification/1 -> Data Type Conversion16/1  "SteerAngle"
  Data Type Conversion5/1 -> Byte Packing 1/6
  Bus Selector1/8 -> Data Type Conversion8/1  "<Omega>"
  Bus Selector1/4 -> Data Type Conversion3/1  "<phi>"
  Cntrl/1 -> Bus Selector2/1
  Data Type Conversion2/1 -> Byte Packing 1/3
  Bus Selector1/10 -> Unit Conversion3/1  "<EngSpd>"
  Unit Conversion1/1 -> Signal Specification1/1
  Bus Selector2/3 -> Unit Conversion2/1  "<SteerCmd>"
  Bus Selector1/3 -> Data Type Conversion2/1  "<GeomZ>"
  Width1/1 -> Send/2
  Bus Selector1/5 -> Data Type Conversion4/1  "<theta>"
  Bus Selector1/7 -> Data Type Conversion7/1  "<dZWheel>"
  Bus Selector2/2 -> Data Type Conversion15/1  "<Brake>"
  Data Type Conversion10/1 -> Byte Packing 1/9
  Bus Selector1/6 -> Data Type Conversion5/1  "<psi>"
  Bus Selector1/9 -> Data Type Conversion10/1  "<WhlAng>"
  Bus Selector1/2 -> Data Type Conversion1/1  "<GeomY>"
  Data Type Conversion7/1 -> Byte Packing 1/7
  Signal Specification1/1 -> Data Type Conversion12/1  "xdot_mph"
  Bus Selector1/1 -> Data Type Conversion6/1  "<GeomX>"
  Data Type Conversion4/1 -> Byte Packing 1/5
  Data Type Conversion6/1 -> Byte Packing 1/1
  Data Type Conversion11/1 -> Byte Packing 1/10
  Data Type Conversion12/1 -> Byte Packing 1/11
  Data Type Conversion13/1 -> Byte Packing 1/12
  Data Type Conversion14/1 -> Byte Packing 1/13
  Data Type Conversion15/1 -> Byte Packing 1/14
  Data Type Conversion16/1 -> Byte Packing 1/15
  [GearCmdVis] -> Data Type Conversion17/1
  [TransmissionModeVis] -> Data Type Conversion9/1
  Data Type Conversion9/1 -> Byte Packing 1/17
  Data Type Conversion17/1 -> Byte Packing 1/16
  Bus Selector/1 -> Mean/1  "<Mz>"
  Mean/1 -> Data Type Conversion18/1
  Data Type Conversion18/1 -> Byte Packing 1/18

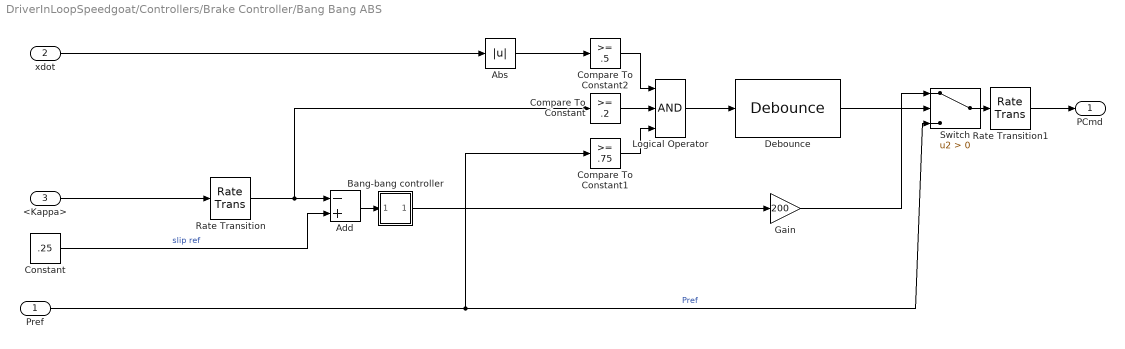
== system DriverInLoopSpeedgoat/Controllers/Brake Controller/Bang Bang ABS ==
  Pref : Inport
  xdot : Inport  Port=2
  <Kappa> : Inport  Port=3
  Abs : Abs
  Add : Sum  Inputs=-+
  Bang-bang controller : Subsystem  mask(Sign){}
      mask help: y = sign(x)
      mask Help: Sign Function:\n\t\t\ty = 1 if x > 0\n\t\t\ty = 0 if x = 0\n\t\t\ty = -1 if x < 0
      mask Display: plot(-50,-50,50,50,[-50,50],[0,0],[0,0],[-50,50],[-40,0],[-30,-30],[0,40],[30,30])
  Compare To Constant : simulink/Logic and Bit Operations/Compare To Constant  relop=>=  const=.2  OutDataTypeStr=boolean
  Compare To Constant1 : simulink/Logic and Bit Operations/Compare To Constant  relop=>=  const=.75  OutDataTypeStr=boolean
  Compare To Constant2 : simulink/Logic and Bit Operations/Compare To Constant  relop=>=  const=.5  OutDataTypeStr=boolean
  Constant : Constant  Value=.25
  Debounce : autolibutils/Debounce  DbcOn_Cnts=.1*.001  DbcOff_Cnts=.1*.001  aMode=aMode
      settings: SourceProductBaseCode=PW,MT,UV,VE,VP
  Gain : Gain  Gain=200
  Logical Operator : Logic  Inputs=3  AllPortsSameDT=off  OutDataTypeStr=boolean
  Rate Transition : RateTransition  OutPortSampleTime=.001
  Rate Transition1 : RateTransition
  Switch : Switch  Criteria=u2 > Threshold  ZeroCross=off
  PCmd : Outport  VectorParamsAs1DForOutWhenUnconnected=off
  wires:
  Bang-bang controller/1(out_1) -> Gain/1
  Add/1 -> Bang-bang controller/1(in_1)
  Rate Transition1/1 -> PCmd/1
  <Kappa>/1 -> Rate Transition/1
  Pref/1 -> Switch/3, Compare To Constant1/1  "Pref"
  Constant/1 -> Add/2  "slip ref"
  Switch/1 -> Rate Transition1/1
  Rate Transition/1 -> Add/1, Compare To Constant/1
  Logical Operator/1 -> Debounce/1
  Compare To Constant/1 -> Logical Operator/2
  Compare To Constant1/1 -> Logical Operator/3
  Debounce/1 -> Switch/2
  xdot/1 -> Abs/1
  Abs/1 -> Compare To Constant2/1
  Compare To Constant2/1 -> Logical Operator/1
  Gain/1 -> Switch/1

== system DriverInLoopSpeedgoat/Controllers/ECU/Rev Limiter Control ==
  TrqCmd : Inport
  EngSpd : Inport  Port=2
  1-D Lookup Table : Lookup_n-D  NumberOfTableDimensions=1  BreakpointsForDimension1=[1 1.01]  Table=[1 0]  ExtrapMethod=Clip  InternalRulePriority=Speed  RndMeth=Simplest  InputSameDT=on
  Constant : Constant  Value=EngRevLim
  Product : Product
  Product1 : Product  Inputs=*/
  TrqCmdRevLimited : Outport  VectorParamsAs1DForOutWhenUnconnected=off
  wires:
  EngSpd/1 -> Product1/1
  Product/1 -> TrqCmdRevLimited/1
  1-D Lookup Table/1 -> Product/2
  TrqCmd/1 -> Product/1
  Constant/1 -> Product1/2
  Product1/1 -> 1-D Lookup Table/1

== system DriverInLoopSpeedgoat/Controllers/Transmission Controller/Automatic ==
  Accel : Inport
  EngSpd : Inport  Port=2  Unit=rad/s
  PrpSpd : Inport  Port=3
  Action Port : ActionPort  ActionPortLabel=case [ 1 ]:
  Neutral Select : Subsystem
  Prop Shaft Speed LPF : DiscreteTransferFcn  Numerator=[0.000000000000000 0.009950166250832 ]  Denominator=[1.000000000000000 -0.990049833749168 ]  mask(DiscretizedDiscreteTransferFcn){}
      mask init:
      | %zoh
  Signal Specification : SignalSpecification  Unit=rpm
  TCM Shift Controller : Stateflow chart  TreatAsAtomicUnit=on
  Unit Conversion : UnitConversion
  prop speed to vehicle speed : Gain  Gain=0.45
  Gear : Outport  VectorParamsAs1DForOutWhenUnconnected=off
  wires:
  TCM Shift Controller/1(GearCmd) -> Gear/1
  Unit Conversion/1 -> Signal Specification/1
  PrpSpd/1 -> Prop Shaft Speed LPF/1
  Signal Specification/1 -> Neutral Select/2(EngSpd)  "EngSpd"
  EngSpd/1 -> Unit Conversion/1
  Accel/1 -> Neutral Select/1(AccCmd), TCM Shift Controller/2(pedal)  "AccCmd"
  Prop Shaft Speed LPF/1 -> prop speed to vehicle speed/1
  prop speed to vehicle speed/1 -> TCM Shift Controller/1(speed)
  Neutral Select/1(Neutral Select) -> TCM Shift Controller/3(Neutral)

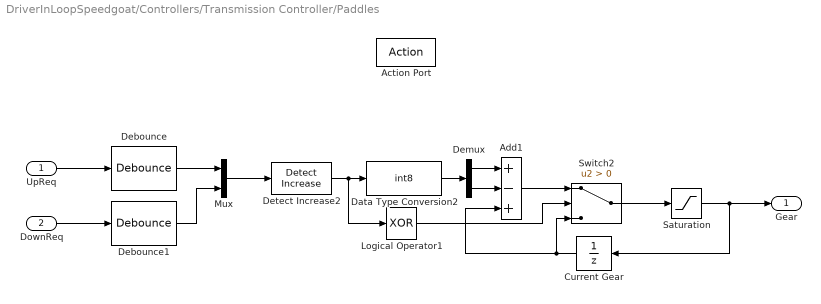
== system DriverInLoopSpeedgoat/Controllers/Transmission Controller/Paddles ==
  UpReq : Inport
  DownReq : Inport  Port=2  Unit=rad/s
  Action Port : ActionPort  ActionPortLabel=case [ 0 ]:
  Add1 : Sum  Inputs=+-+
  Current Gear : UnitDelay  SampleTime=-1  HasFrameUpgradeWarning=on
  Data Type Conversion2 : DataTypeConversion  OutDataTypeStr=int8
  Debounce : autolibutils/Debounce  DbcOn_Cnts=10  DbcOff_Cnts=10  aMode=aMode
      settings: SourceProductBaseCode=PW,MT,UV,VE,VP
  Debounce1 : autolibutils/Debounce  DbcOn_Cnts=10  DbcOff_Cnts=10  aMode=aMode
      settings: SourceProductBaseCode=PW,MT,UV,VE,VP
  Demux : Demux  Outputs=2
  Detect Increase2 : simulink/Logic and Bit Operations/Detect Increase  vinit=0.0  OutDataTypeStr=boolean
  Logical Operator1 : Logic  Operator=XOR  Inputs=1  AllPortsSameDT=off  OutDataTypeStr=boolean
  Mux : Mux  Inputs=2
  Saturation : Saturate  UpperLimit=5  LowerLimit=-1
  Switch2 : Switch  Criteria=u2 > Threshold
  Gear : Outport  VectorParamsAs1DForOutWhenUnconnected=off
  wires:
  Saturation/1 -> Gear/1, Current Gear/1
  UpReq/1 -> Debounce/1
  Current Gear/1 -> Add1/3, Switch2/3
  Debounce1/1 -> Mux/2
  Data Type Conversion2/1 -> Demux/1
  Add1/1 -> Switch2/1
  Mux/1 -> Detect Increase2/1
  Detect Increase2/1 -> Data Type Conversion2/1, Logical Operator1/1
  Logical Operator1/1 -> Switch2/2
  Debounce/1 -> Mux/1
  DownReq/1 -> Debounce1/1
  Demux/2 -> Add1/2
  Demux/1 -> Add1/1
  Switch2/1 -> Saturation/1

== system DriverInLoopSpeedgoat/Environment/Friction Scaling/Constant ==
  Bus Creator2 : BusCreator  Inputs=4
  Constant Mu : Constant  Value=ones(4,1).*1.5
  Demux1 : Demux
  Signal Specification1 : SignalSpecification  Unit=1
  mu : Outport  VectorParamsAs1DForOutWhenUnconnected=off
  wires:
  Demux1/3 -> Bus Creator2/3  "mu_RL"
  Demux1/4 -> Bus Creator2/4  "mu_RR"
  Demux1/1 -> Bus Creator2/1  "mu_FL"
  Demux1/2 -> Bus Creator2/2  "mu_FR"
  Bus Creator2/1 -> mu/1  "mu"
  Constant Mu/1 -> Signal Specification1/1
  Signal Specification1/1 -> Demux1/1

== system DriverInLoopSpeedgoat/Environment/Friction Scaling/Lookup Table ==
  VehFdbk : Inport
  Bus Creator2 : BusCreator  Inputs=4
  Bus Creator3 : BusCreator  Inputs=1
  Bus Selector : BusSelector  OutputSignals=Wheels.XWheel,Wheels.YWheel
  Demux1 : Demux
  Memory : Memory
  Memory1 : Memory
  Split Mu : Subsystem  TreatAsAtomicUnit=on
  mu : Outport  VectorParamsAs1DForOutWhenUnconnected=off
  wires:
  Demux1/1 -> Bus Creator2/1  "mu_FL"
  Demux1/3 -> Bus Creator2/3  "mu_RL"
  Demux1/4 -> Bus Creator2/4  "mu_RR"
  Demux1/2 -> Bus Creator2/2  "mu_FR"
  Bus Creator2/1 -> Bus Creator3/1  "mu"
  Bus Creator3/1 -> mu/1
  Memory/1 -> Split Mu/1(In1)
  Bus Selector/1 -> Memory/1  "<XWheel>"
  Memory1/1 -> Split Mu/2(In2)
  Bus Selector/2 -> Memory1/1  "<YWheel>"
  VehFdbk/1 -> Bus Selector/1
  Split Mu/1(Out1) -> Demux1/1

== system DriverInLoopSpeedgoat/Environment/Ground Height/3D Engine ==
  Bus Creator : BusCreator  Inputs=4
  Data Type Conversion : DataTypeConversion
  Data Type Conversion1 : DataTypeConversion  OutDataTypeStr=boolean
  Demux : Demux
  Signal Specification : SignalSpecification  Unit=m
  Subsystem : Subsystem
  While Iterator Subsystem : Subsystem  TreatAsAtomicUnit=on
  z : Outport  VectorParamsAs1DForOutWhenUnconnected=off
  wires:
  Demux/2 -> Bus Creator/2  "G_FR_z"
  Demux/1 -> Bus Creator/1  "G_FL_z"
  Demux/4 -> Bus Creator/4  "G_RR_z"
  Demux/3 -> Bus Creator/3  "G_RL_z"
  Bus Creator/1 -> z/1  "z"
  Data Type Conversion/1 -> Signal Specification/1
  Signal Specification/1 -> Demux/1
  Subsystem/1(Rx Data) -> Data Type Conversion/1
  While Iterator Subsystem/1(Data) -> Subsystem/1(In1)
  Data Type Conversion1/1 -> Subsystem/Enable
  While Iterator Subsystem/2(NumMsg) -> Data Type Conversion1/1

== system DriverInLoopSpeedgoat/Environment/Ground Height/Constant ==
  Bus Creator : BusCreator  Inputs=4
  Bus Creator3 : BusCreator  Inputs=1
  Constant1 : Constant  Value=zeros(4,1)
  Demux : Demux
  Signal Specification : SignalSpecification  Unit=m
  z : Outport  VectorParamsAs1DForOutWhenUnconnected=off
  wires:
  Constant1/1 -> Signal Specification/1
  Signal Specification/1 -> Demux/1
  Demux/4 -> Bus Creator/4  "G_RR_z"
  Demux/1 -> Bus Creator/1  "G_FL_z"
  Demux/3 -> Bus Creator/3  "G_RL_z"
  Demux/2 -> Bus Creator/2  "G_FR_z"
  Bus Creator/1 -> Bus Creator3/1  "z"
  Bus Creator3/1 -> z/1

== system DriverInLoopSpeedgoat/External Driver Input/External Driver - Host/Receive UDP ==
  Compare To Constant : simulink/Logic and Bit Operations/Compare To Constant  relop===  const=19  OutDataTypeStr=boolean
  Constant : Constant  OutDataTypeStr=Inherit: Inherit via back propagation  SampleTime=-1
  Receive : slrealtimeiplib/UDP Receive  useHostTargetConn=on  ipAddress=target_ip  localPort=25003  rcvWidth=19  rcvFmAny=off  fmAddress=host_ip  rcvMulticast=off  multicastAddress=[]  sampleTime=-1
      settings: SourceProductBaseCode=XP
  Subtract : Sum  Inputs=+-
  While Iterator : WhileIterator  MaxIters=10  WhileBlockType=do-while  ShowIterationPort=on
  NumMsg : Outport
  Data : Outport  Port=2
  wires:
  Receive/2 -> Compare To Constant/1
  Compare To Constant/1 -> While Iterator/1
  While Iterator/1 -> Subtract/1
  Constant/1 -> Subtract/2
  Receive/1 -> Data/1
  Subtract/1 -> NumMsg/1

== system DriverInLoopSpeedgoat/External Driver Input/External Driver - Host/Subsystem ==
  In1 : Inport
  Enable : EnablePort
  Byte Unpacking : slrealtimeutilitieslib/Byte Unpacking  MaskUnpackedDataTypes={'double','double','boolean','boolean','boolean'}  MaskUnpackedDataSizes={[1],[1],[1],[1],[1]}  MaskAlignment=1
      settings: SourceProductBaseCode=XP
  Steer : Outport
  AccelBrake : Outport  Port=2
  ShiftDn : Outport  Port=3
  ShiftUp : Outport  Port=4
  ToggleMode : Outport  Port=5
  wires:
  In1/1 -> Byte Unpacking/1
  Byte Unpacking/2 -> AccelBrake/1  "AccelBrake"
  Byte Unpacking/3 -> ShiftDn/1  "ShiftDn"
  Byte Unpacking/4 -> ShiftUp/1  "ShiftUp"
  Byte Unpacking/1 -> Steer/1  "Steer"
  Byte Unpacking/5 -> ToggleMode/1  "Toggle"

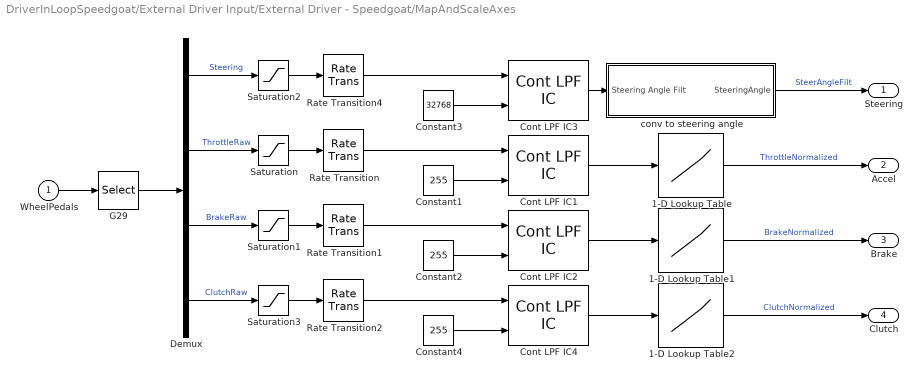
== system DriverInLoopSpeedgoat/External Driver Input/External Driver - Speedgoat/MapAndScaleAxes ==
  WheelPedals : Inport
  1-D Lookup Table : Lookup_n-D  NumberOfTableDimensions=1  BreakpointsForDimension1=[0 255]  Table=[1 0]  ExtrapMethod=Clip  UseLastTableValue=on  InternalRulePriority=Speed  RndMeth=Simplest  InputSameDT=on
  1-D Lookup Table1 : Lookup_n-D  NumberOfTableDimensions=1  BreakpointsForDimension1=[0 255]  Table=[1 0]  ExtrapMethod=Clip  UseLastTableValue=on  InternalRulePriority=Speed  RndMeth=Simplest  InputSameDT=on
  1-D Lookup Table2 : Lookup_n-D  NumberOfTableDimensions=1  BreakpointsForDimension1=[0 255]  Table=[1 0]  ExtrapMethod=Clip  UseLastTableValue=on  InternalRulePriority=Speed  RndMeth=Simplest  InputSameDT=on
  Constant1 : Constant  Value=255
  Constant2 : Constant  Value=255
  Constant3 : Constant  Value=32768
  Constant4 : Constant  Value=255
  Cont LPF IC1 : autolibutils/Cont LPF IC  wc=8*pi  aMode=aMode  dataType=off
      settings: SourceProductBaseCode=PW,MT,UV,VE,VP
  Cont LPF IC2 : autolibutils/Cont LPF IC  wc=8*pi  aMode=aMode  dataType=off
      settings: SourceProductBaseCode=PW,MT,UV,VE,VP
  Cont LPF IC3 : autolibutils/Cont LPF IC  wc=10  aMode=aMode  dataType=off
      settings: SourceProductBaseCode=PW,MT,UV,VE,VP
  Cont LPF IC4 : autolibutils/Cont LPF IC  wc=8*pi  aMode=aMode  dataType=off
      settings: SourceProductBaseCode=PW,MT,UV,VE,VP
  Demux : Demux
  G29 : Selector  InputPortWidth=4  IndexOptions=Index vector (dialog)  Indices=[1 2 3 4]  OutputSizes=1
  Rate Transition : RateTransition  Integrity=off  InitialCondition=4095
  Rate Transition1 : RateTransition  Integrity=off  InitialCondition=4095
  Rate Transition2 : RateTransition  Integrity=off  InitialCondition=4095
  Rate Transition4 : RateTransition  Integrity=off  Deterministic=off  InitialCondition=4095
  Saturation : Saturate  UpperLimit=255  LowerLimit=0
  Saturation1 : Saturate  UpperLimit=255  LowerLimit=0
  Saturation2 : Saturate  UpperLimit=65535  LowerLimit=0
  Saturation3 : Saturate  UpperLimit=4096  LowerLimit=0
  conv to steering angle : Subsystem
  Steering : Outport  VectorParamsAs1DForOutWhenUnconnected=off
  Accel : Outport  Port=2  VectorParamsAs1DForOutWhenUnconnected=off
  Brake : Outport  Port=3  VectorParamsAs1DForOutWhenUnconnected=off
  Clutch : Outport  Port=4  VectorParamsAs1DForOutWhenUnconnected=off
  wires:
  WheelPedals/1 -> G29/1
  1-D Lookup Table2/1 -> Clutch/1  "ClutchNormalized"
  conv to steering angle/1(SteeringAngle) -> Steering/1  "SteerAngleFilt"
  Constant2/1 -> Cont LPF IC2/2
  Constant3/1 -> Cont LPF IC3/2
  Demux/2 -> Saturation/1  "ThrottleRaw"
  Demux/1 -> Saturation2/1  "Steering"
  Cont LPF IC2/1 -> 1-D Lookup Table1/1
  Demux/4 -> Saturation3/1  "ClutchRaw"
  1-D Lookup Table/1 -> Accel/1  "ThrottleNormalized"
  Cont LPF IC1/1 -> 1-D Lookup Table/1
  Cont LPF IC4/1 -> 1-D Lookup Table2/1
  Demux/3 -> Saturation1/1  "BrakeRaw"
  1-D Lookup Table1/1 -> Brake/1  "BrakeNormalized"
  Constant1/1 -> Cont LPF IC1/2
  Constant4/1 -> Cont LPF IC4/2
  G29/1 -> Demux/1
  Saturation3/1 -> Rate Transition2/1
  Saturation1/1 -> Rate Transition1/1
  Saturation/1 -> Rate Transition/1
  Saturation2/1 -> Rate Transition4/1
  Rate Transition/1 -> Cont LPF IC1/1
  Rate Transition1/1 -> Cont LPF IC2/1
  Rate Transition2/1 -> Cont LPF IC4/1
  Rate Transition4/1 -> Cont LPF IC3/1
  Cont LPF IC3/1 -> conv to steering angle/1(Steering Angle Filt)

== system DriverInLoopSpeedgoat/External Driver Input/External Driver - Speedgoat/MapButtons ==
  Buttons : Inport
  Data Type Conversion : DataTypeConversion
  Data Type Conversion1 : DataTypeConversion
  Demux3 : Demux  Outputs=2
  G29 : Selector  InputPortWidth=13  IndexOptions=Index vector (dialog)  Indices=[5 6 1 2 3 4 7 8 9 10 11 12 13]  OutputSizes=1
  Select Left and Right Shift Paddle buttons : Selector  InputPortWidth=13  IndexOptions=Index vector (dialog)  Indices=[1 2]  OutputSizes=1
  LeftPaddle : Outport  VectorParamsAs1DForOutWhenUnconnected=off
  RightPaddle : Outport  Port=2  VectorParamsAs1DForOutWhenUnconnected=off
  AllButtons : Outport  Port=3  VectorParamsAs1DForOutWhenUnconnected=off
  wires:
  Buttons/1 -> G29/1
  Data Type Conversion/1 -> LeftPaddle/1
  Data Type Conversion1/1 -> RightPaddle/1
  Demux3/1 -> Data Type Conversion/1  "Left Paddle"
  Demux3/2 -> Data Type Conversion1/1  "Right Paddle"
  Select Left and Right Shift Paddle buttons/1 -> Demux3/1
  G29/1 -> AllButtons/1, Select Left and Right Shift Paddle buttons/1

== system DriverInLoopSpeedgoat/Controllers/Brake Controller/Bang Bang ABS/Bang-bang controller ==
  in_1 : Inport
  Constant : Constant  Value=0
  Data Type Conversion1 : DataTypeConversion  OutDataTypeStr=double  SaturateOnIntegerOverflow=on  RndMeth=Zero
  Data Type Conversion2 : DataTypeConversion  OutDataTypeStr=double  SaturateOnIntegerOverflow=on  RndMeth=Zero
  Relational Operator : RelationalOperator  Operator=>  OutDataTypeStr=boolean  RndMeth=Nearest  InputSameDT=on
  Relational Operator1 : RelationalOperator  Operator=<  OutDataTypeStr=boolean  RndMeth=Nearest  InputSameDT=on
  Sum : Sum  Inputs=+-  InputSameDT=on  SaturateOnIntegerOverflow=on  OutDataTypeStr=Inherit: Same as first input
  out_1 : Outport  VectorParamsAs1DForOutWhenUnconnected=off
  wires:
  Data Type Conversion2/1 -> Sum/2
  Data Type Conversion1/1 -> Sum/1
  Sum/1 -> out_1/1
  Relational Operator/1 -> Data Type Conversion1/1
  Relational Operator1/1 -> Data Type Conversion2/1
  Constant/1 -> Relational Operator/2, Relational Operator1/2
  in_1/1 -> Relational Operator1/1, Relational Operator/1

== system DriverInLoopSpeedgoat/Controllers/Transmission Controller/Automatic/Neutral Select ==
  AccCmd : Inport
  EngSpd : Inport  Port=2
  Constant : Constant  Value=1200
  Constant1 : Constant  Value=1e-6
  Logical Operator : Logic  AllPortsSameDT=off  OutDataTypeStr=boolean
  Relational Operator : RelationalOperator  Operator=<=  OutDataTypeStr=boolean  RndMeth=Simplest
  Relational Operator1 : RelationalOperator  Operator=<=  OutDataTypeStr=boolean  RndMeth=Simplest
  Neutral Select : Outport  VectorParamsAs1DForOutWhenUnconnected=off
  wires:
  EngSpd/1 -> Relational Operator/1
  Relational Operator1/1 -> Logical Operator/1
  AccCmd/1 -> Relational Operator1/1
  Constant1/1 -> Relational Operator1/2
  Logical Operator/1 -> Neutral Select/1
  Constant/1 -> Relational Operator/2
  Relational Operator/1 -> Logical Operator/2
